simulink model "SINDM"  (R2021a)
settings: Solver=VariableStepAuto  StartTime=0.0  StopTime=10.0  RelTol=1e-3
libraries: dsparch4 x2, dspquant2 x2
settings Model: Creator=RUKU  LastModifiedBy=RUKU

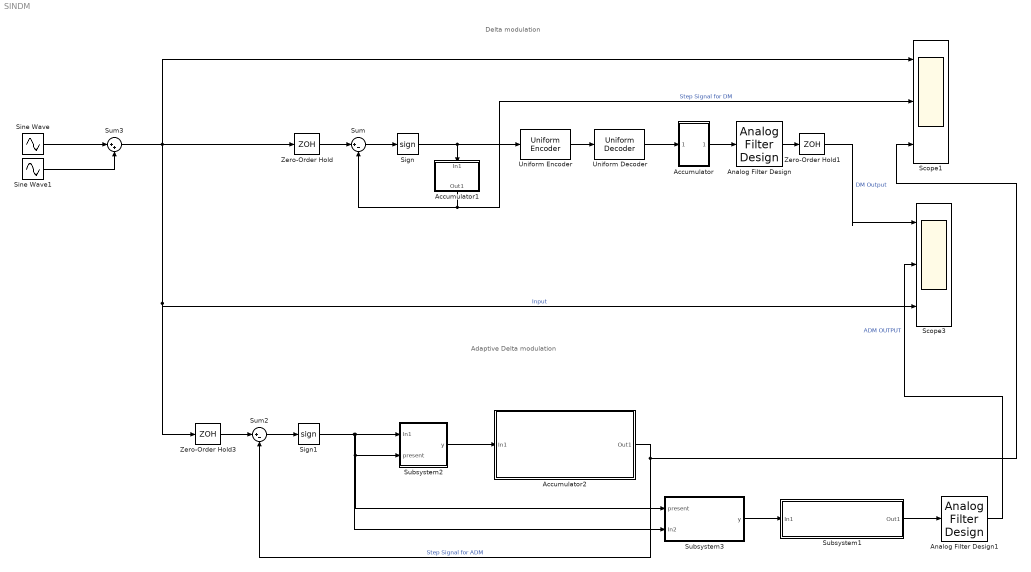
== system SINDM ==
  note: Adaptive Delta modulation
  note: Delta modulation
  Accumulator : Subsystem
  Accumulator1 : Subsystem
  Accumulator2 : Subsystem
  Analog Filter Design : dsparch4/Analog Filter Design  method=Butterworth  filttype=Lowpass  N=8  Wlo=2*pi*600  Whi=80  Rp=2  Rs=40
  Analog Filter Design1 : dsparch4/Analog Filter Design  method=Butterworth  filttype=Lowpass  N=8  Wlo=2*pi*600  Whi=80  Rp=2  Rs=40
  Scope1 : Scope  NumInputPorts=3
  Scope3 : Scope  NumInputPorts=3
  Sign : Signum
  Sign1 : Signum
  Sine Wave : Sin  Frequency=2*pi*100  SampleTime=0
  Sine Wave1 : Sin  Frequency=2*pi*200  SampleTime=0
  Subsystem1 : Subsystem
  Subsystem2 : Subsystem
  Subsystem3 : Subsystem
  Sum : Sum  Inputs=|+-
  Sum2 : Sum  Inputs=|+-
  Sum3 : Sum  Inputs=|++
  Uniform Decoder : dspquant2/Uniform Decoder  peak=2  bits=16  overflowMode=Saturate  otype=Double
      settings: SourceProductBaseCode=DS
  Uniform Encoder : dspquant2/Uniform Encoder  peak=2  bits=16  otype=Signed integer
  Zero-Order Hold : ZeroOrderHold  SampleTime=1/16000
  Zero-Order Hold1 : ZeroOrderHold  SampleTime=1/16000
  Zero-Order Hold3 : ZeroOrderHold  SampleTime=1/16000
  wires:
  Sum3/1 -> Zero-Order Hold/1, Scope3/3, Zero-Order Hold3/1, Scope1/1  "Input"
  Zero-Order Hold3/1 -> Sum2/1
  Analog Filter Design1/1 -> Scope3/2  "ADM OUTPUT"
  Sum2/1 -> Sign1/1
  Subsystem3/1(y) -> Subsystem1/1(In1)
  Sign1/1 -> Subsystem2/1(In1), Subsystem3/1(present), Subsystem2/2(present), Subsystem3/2(In2)
  Zero-Order Hold/1 -> Sum/1
  Analog Filter Design/1 -> Zero-Order Hold1/1
  Subsystem1/1(Out1) -> Analog Filter Design1/1
  Uniform Decoder/1 -> Accumulator/1(In1)
  Uniform Encoder/1 -> Uniform Decoder/1
  Accumulator/1(Out1) -> Analog Filter Design/1
  Zero-Order Hold1/1 -> Scope3/1  "DM Output"
  Accumulator1/1(Out1) -> Sum/2, Scope1/2  "Step Signal for DM"
  Subsystem2/1(y) -> Accumulator2/1(In1)
  Accumulator2/1(Out1) -> Sum2/2, Scope1/3  "Step Signal for ADM"
  Sum/1 -> Sign/1
  Sign/1 -> Uniform Encoder/1, Accumulator1/1(In1)
  Sine Wave/1 -> Sum3/1
  Sine Wave1/1 -> Sum3/2

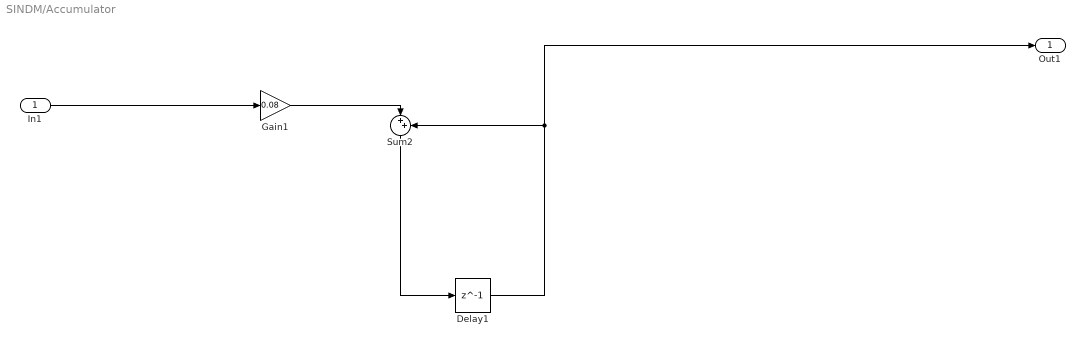
== system SINDM/Accumulator ==
  In1 : Inport
  Delay1 : Delay  DelayLength=1
  Gain1 : Gain  Gain=0.08
  Sum2 : Sum  Inputs=|++
  Out1 : Outport
  wires:
  In1/1 -> Gain1/1
  Delay1/1 -> Out1/1, Sum2/2
  Sum2/1 -> Delay1/1
  Gain1/1 -> Sum2/1

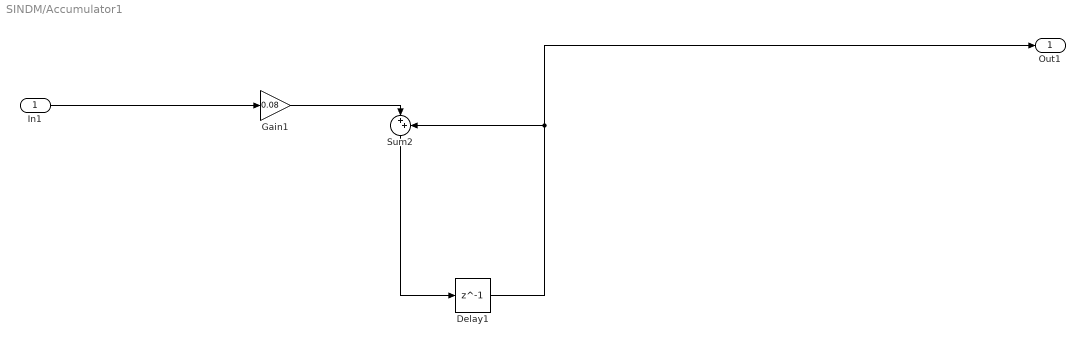
== system SINDM/Accumulator1 ==
  In1 : Inport
  Delay1 : Delay  DelayLength=1
  Gain1 : Gain  Gain=0.08
  Sum2 : Sum  Inputs=|++
  Out1 : Outport
  wires:
  In1/1 -> Gain1/1
  Delay1/1 -> Out1/1, Sum2/2
  Sum2/1 -> Delay1/1
  Gain1/1 -> Sum2/1

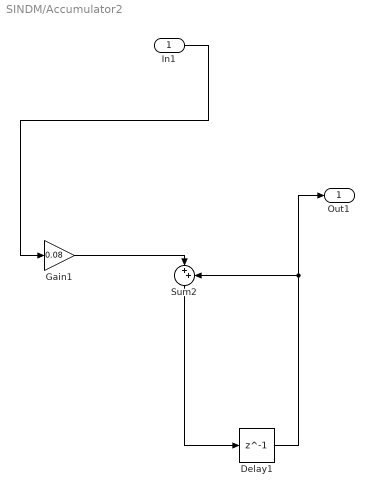
== system SINDM/Accumulator2 ==
  In1 : Inport
  Delay1 : Delay  DelayLength=1
  Gain1 : Gain  Gain=0.08
  Sum2 : Sum  Inputs=|++
  Out1 : Outport
  wires:
  Delay1/1 -> Out1/1, Sum2/2
  Gain1/1 -> Sum2/1
  Sum2/1 -> Delay1/1
  In1/1 -> Gain1/1

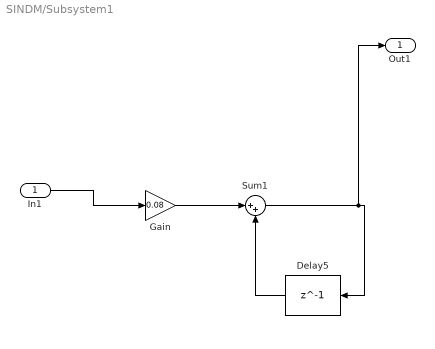
== system SINDM/Subsystem1 ==
  In1 : Inport
  Delay5 : Delay  DelayLength=1  InputProcessing=Columns as channels (frame based)
  Gain : Gain  Gain=0.08
  Sum1 : Sum  Inputs=|++
  Out1 : Outport
  wires:
  Delay5/1 -> Sum1/2
  Sum1/1 -> Out1/1, Delay5/1
  Gain/1 -> Sum1/1
  In1/1 -> Gain/1

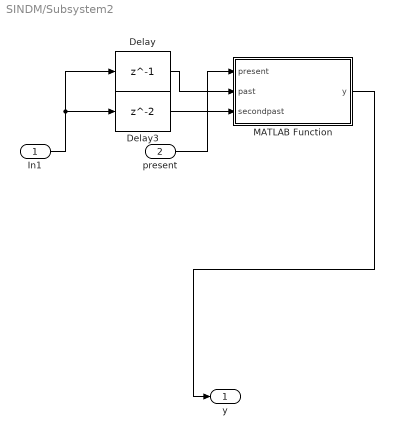
== system SINDM/Subsystem2 ==
  In1 : Inport
  present : Inport  Port=2
  Delay : Delay  DelayLength=1  InputProcessing=Columns as channels (frame based)
  Delay3 : Delay  InputProcessing=Columns as channels (frame based)
  MATLAB Function : MATLAB Function  TreatAsAtomicUnit=on
  y : Outport
  wires:
  In1/1 -> Delay3/1, Delay/1
  present/1 -> MATLAB Function/1(present)
  Delay3/1 -> MATLAB Function/3(secondpast)
  Delay/1 -> MATLAB Function/2(past)
  MATLAB Function/1(y) -> y/1

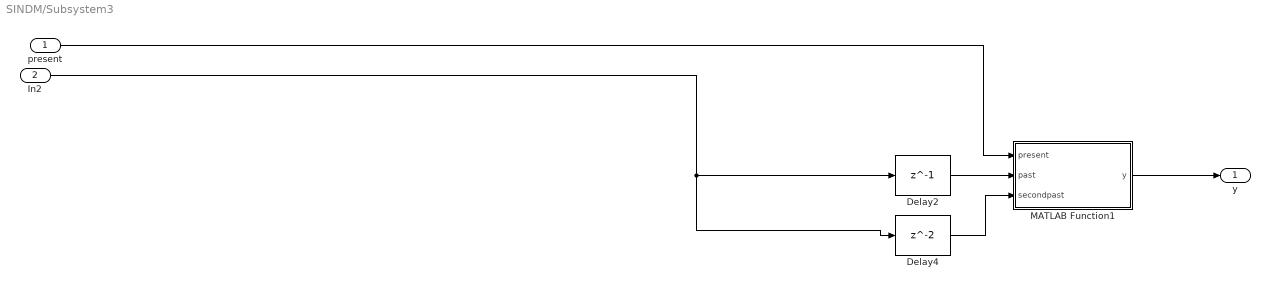
== system SINDM/Subsystem3 ==
  present : Inport
  In2 : Inport  Port=2
  Delay2 : Delay  DelayLength=1  InputProcessing=Columns as channels (frame based)
  Delay4 : Delay  InputProcessing=Columns as channels (frame based)
  MATLAB Function1 : MATLAB Function  TreatAsAtomicUnit=on
  y : Outport
  wires:
  present/1 -> MATLAB Function1/1(present)
  Delay2/1 -> MATLAB Function1/2(past)
  In2/1 -> Delay4/1, Delay2/1
  MATLAB Function1/1(y) -> y/1
  Delay4/1 -> MATLAB Function1/3(secondpast)

== matlab function SINDM/Subsystem2/MATLAB Function ==
  data: present input; y output; past input; secondpast input
function y = control(present,past,secondpast)

if present == past 
    if present == secondpast
        y=4*present;
    else
        y=2*present;
    end
else
    y=1*present;
    
end
end

== matlab function SINDM/Subsystem3/MATLAB Function1 ==
  data: present input; y output; past input; secondpast input
function y = control(present,past,secondpast)

if present == past 
    if present == secondpast
        y=4*present;
    else
        y=2*present;
    end
else
    y=1*present;
    
end
end
